simulink library "casper_library"  (Simulink 6.5)
PostLoadFcn:
  | % Stub definitions for mask variables
  | delay_depth=16;
  | n_bits=8;
  | bin_pt=7;
values from neighbouring files (symbols this model uses):
  add_latency = get_var('add_latency', 'defaults', defaults, varargin{:})    [butterfly_direct_init.m]    (also in fft_direct_init.m; fft_init.m; fft_wideband_real_init.m; pfb_real_add_tree_init.m)
  BitWidthIn = get_var('BitWidthIn', 'defaults', defaults, varargin{:})    [pfb_real_add_tree_init.m]
  blockCountBits = ceil(log2(numBlocks))    [address_gen_vacc_v2_mask.m]
  blockRowBits = 0    [address_gen_vacc_v2_mask.m]
  CoeffBitWidth = get_var('CoeffBitWidth', 'defaults', defaults, varargin{:})    [pfb_coeff_gen_init.m]    (also in pfb_real_add_tree_init.m)
  mult_latency = get_var('mult_latency', 'defaults', defaults, varargin{:})    [butterfly_direct_init.m]    (also in fft_direct_init.m; fft_init.m; fft_wideband_real_init.m)
  n_inputs = get_var('n_inputs', 'defaults', defaults, varargin{:})    [fft_init.m]    (also in fft_unscrambler_init.m; fft_wideband_real_init.m; partial_delay_init.m = get_var('n_inputs', varargin{:}); pfb_coeff_gen_init.m)
  PFBSize = get_var('PFBSize', 'defaults', defaults, varargin{:})    [pfb_coeff_gen_init.m]
undefined symbols (not defined in the file or in its folder): acc_len, ant_bits, bit_growth, cmult_4bit_br, cmult_4bit_em, cmult_4bit_sl, n_ants, n_bits_out, num_ants
libraries: xbsIndex_r3 x1646, xbsIndex_r4 x226, casper_library x156, xbsReplacements_r4 x17, xps_library x10, fft_library x4
(part 7 of 14)

== system casper_library/Correlator/x_engine_reorder/win2_ctrl ==
  write : Inport
  win_valid : Inport  Port=2
  sync : Inport  Port=3
  Constant : xbsIndex_r3/Constant  const=num_elements  equ=P=C  arith_type=Unsigned  n_bits=elements_bits + 1  bin_pt=0  opselect=C  inp2=PCIN>>17  opr=+  inp1=P  carry=CIN  iostate=0  explicit_period=on  period=1  dbl_ovrd=off
  Constant1 : xbsIndex_r3/Constant  const=num_elements * 2 - 2  equ=P=C  arith_type=Unsigned  n_bits=elements_bits + 1  bin_pt=0  opselect=C  inp2=PCIN>>17  opr=+  inp1=P  carry=CIN  iostate=0  explicit_period=on  period=1  dbl_ovrd=off
  Constant3 : xbsIndex_r3/Constant  const=num_elements * 2 - 1  equ=P=C  arith_type=Unsigned  n_bits=elements_bits + 1  bin_pt=0  opselect=C  inp2=PCIN>>17  opr=+  inp1=P  carry=CIN  iostate=0  explicit_period=on  period=1  dbl_ovrd=off
  Constant6 : xbsIndex_r3/Constant  const=num_elements  equ=P=C  arith_type=Unsigned  n_bits=elements_bits + 1  bin_pt=0  opselect=C  inp2=PCIN>>17  opr=+  inp1=P  carry=CIN  iostate=0  explicit_period=on  period=1  dbl_ovrd=off
  Counter : xbsIndex_r3/Counter  cnt_type=Free Running  n_bits=elements_bits + 1  bin_pt=0  arith_type=Unsigned  start_count=num_elements * 2 - 1 - addr_offset  cnt_to=71  cnt_by_val=1  operation=Up  explicit_period=off  period=1  load_pin=on  rst=on  en=on  dbl_ovrd=off  show_param=off  use_rpm=on  gen_core=off
      settings: xl_area=[0, 0, 0, 0, 0, 0, 0]
  Delay10 : xbsIndex_r3/Delay  latency=1  reg_retiming=off  explicit_period=off  period=1  en=on  accept_only_valid=off  init_zero=on  dbl_ovrd=off  show_param=off
      settings: xl_area=[0, 0, 0, 0, 0, 0, 0]
  Delay12 : xbsIndex_r3/Delay  latency=1  reg_retiming=off  explicit_period=off  period=1  en=on  accept_only_valid=off  init_zero=on  dbl_ovrd=off  show_param=off
      settings: xl_area=[0, 0, 0, 0, 0, 0, 0]
  Logical3 : xbsIndex_r3/Logical  logical_function=AND  inputs=2  precision=Full  arith_type=Unsigned  n_bits=8  bin_pt=2  align_bp=on  latency=0  explicit_period=off  period=1  en=off  dbl_ovrd=off  show_param=off
      settings: xl_area=[0, 0, 0, 0, 0, 0, 0]
  Logical6 : xbsIndex_r3/Logical  logical_function=AND  inputs=2  precision=Full  arith_type=Unsigned  n_bits=8  bin_pt=2  align_bp=on  latency=0  explicit_period=off  period=1  en=off  dbl_ovrd=off  show_param=off
      settings: xl_area=[0, 0, 0, 0, 0, 0, 0]
  Relational : xbsIndex_r3/Relational  mode=a>=b  latency=1  explicit_period=on  period=1  en=off  dbl_ovrd=off  show_param=off
      settings: xl_area=[0, 0, 0, 0, 0, 0, 0]
  Relational2 : xbsIndex_r3/Relational  mode=a=b  latency=1  explicit_period=on  period=1  en=off  dbl_ovrd=off  show_param=off
      settings: xl_area=[0, 0, 0, 0, 0, 0, 0]
  Relational4 : xbsIndex_r3/Relational  mode=a=b  latency=1  explicit_period=on  period=1  en=off  dbl_ovrd=off  show_param=off
      settings: xl_area=[0, 0, 0, 0, 0, 0, 0]
  pulse_extender1 : Subsystem  mask{num_elements=num_elements}
      mask prompts: num_elements "Length of Pulse"
      mask init:
      | pulse_len = 2*num_elements;
      | bits = ceil(log2(pulse_len));
  write_addr : Outport
  read : Outport  Port=2
  read_valid : Outport  Port=3
  wires:
  Constant/1 -> Counter/2
  Constant1/1 -> Relational/2
  Counter/1 -> Relational/1, Relational2/1, Relational4/1, write_addr/1
  Relational/1 -> Counter/1
  pulse_extender1/1(out) -> Logical6/1, read/1
  Constant3/1 -> Relational2/2
  Relational2/1 -> pulse_extender1/1(in), Delay12/2
  Constant6/1 -> Relational4/2
  Relational4/1 -> Logical3/1
  Logical3/1 -> Delay10/2
  Delay10/1 -> Delay12/1
  Delay12/1 -> Logical6/2
  sync/1 -> Counter/3
  win_valid/1 -> Delay10/1
  write/1 -> Counter/4, Logical3/2
  Logical6/1 -> read_valid/1

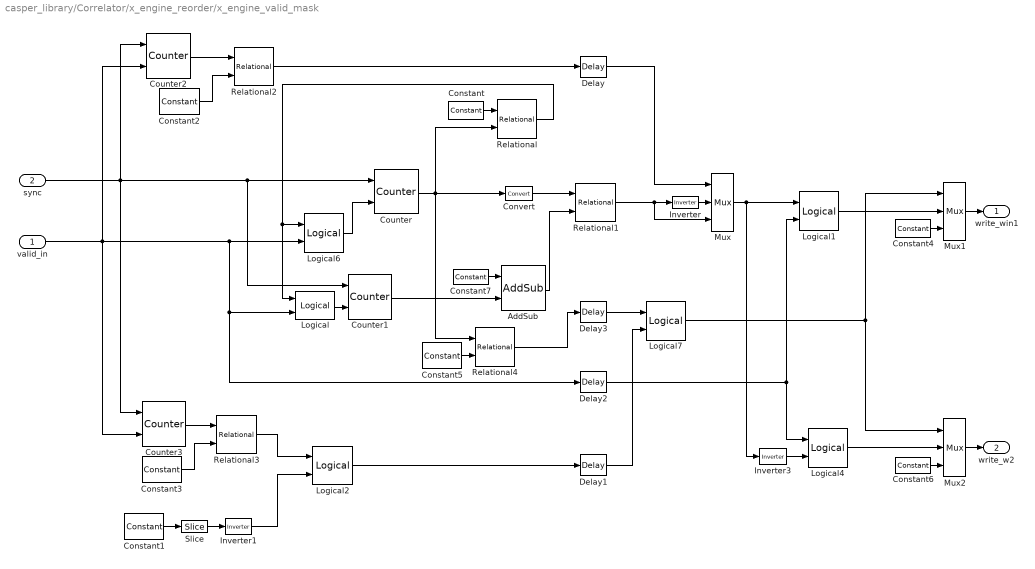
== system casper_library/Correlator/x_engine_reorder/x_engine_valid_mask ==
  valid_in : Inport
  sync : Inport  Port=2
  AddSub : xbsIndex_r3/AddSub  mode=Subtraction  precision=Full  arith_type=Unsigned  n_bits=8  bin_pt=2  quantization=Truncate  overflow=Wrap  latency=0  explicit_period=off  period=1  use_carryin=off  use_carryout=off  en=off  dbl_ovrd=off  show_param=off  use_core=on  pipeline=off  use_rpm=on  gen_core=off
      settings: xl_area=[0, 0, 0, 0, 0, 0, 0]
  Constant : xbsIndex_r3/Constant  const=num_taps-1  equ=P=C  arith_type=Unsigned  n_bits=cntr_bits  bin_pt=0  opselect=C  inp2=PCIN>>17  opr=+  inp1=P  carry=CIN  iostate=0  explicit_period=on  period=1  dbl_ovrd=off
  Constant1 : xbsIndex_r3/Constant  const=num_ants  equ=P=C  arith_type=Unsigned  n_bits=ant_bits  bin_pt=0  opselect=C  inp2=PCIN>>17  opr=+  inp1=P  carry=CIN  iostate=0  explicit_period=on  period=1  dbl_ovrd=off
  Constant2 : xbsIndex_r3/Constant  const=num_validins  equ=P=C  arith_type=Unsigned  n_bits=validin_bits  bin_pt=0  opselect=C  inp2=PCIN>>17  opr=+  inp1=P  carry=CIN  iostate=0  explicit_period=on  period=1  dbl_ovrd=off
  Constant3 : xbsIndex_r3/Constant  const=num_validins/2  equ=P=C  arith_type=Unsigned  n_bits=validin_bits - 1  bin_pt=0  opselect=C  inp2=PCIN>>17  opr=+  inp1=P  carry=CIN  iostate=0  explicit_period=on  period=1  dbl_ovrd=off
  Constant4 : xbsIndex_r3/Constant  const=0  equ=P=C  arith_type=Boolean  n_bits=1  bin_pt=0  opselect=C  inp2=PCIN>>17  opr=+  inp1=P  carry=CIN  iostate=0  explicit_period=on  period=1  dbl_ovrd=off
  Constant5 : xbsIndex_r3/Constant  const=0  equ=P=C  arith_type=Unsigned  n_bits=cntr_bits  bin_pt=0  opselect=C  inp2=PCIN>>17  opr=+  inp1=P  carry=CIN  iostate=0  explicit_period=on  period=1  dbl_ovrd=off
  Constant6 : xbsIndex_r3/Constant  const=0  equ=P=C  arith_type=Boolean  n_bits=1  bin_pt=0  opselect=C  inp2=PCIN>>17  opr=+  inp1=P  carry=CIN  iostate=0  explicit_period=on  period=1  dbl_ovrd=off
  Constant7 : xbsIndex_r3/Constant  const=num_taps-1  equ=P=C  arith_type=Unsigned  n_bits=cntr_bits  bin_pt=0  opselect=C  inp2=PCIN>>17  opr=+  inp1=P  carry=CIN  iostate=0  explicit_period=on  period=1  dbl_ovrd=off
  Convert : xbsIndex_r3/Convert  arith_type=Unsigned  n_bits=cntr_bits+1  bin_pt=0  quantization=Truncate  overflow=Wrap  latency=0  explicit_period=off  period=1  dbl_ovrd=off  show_param=off  inserted_by_tool=off  pipeline=off
      settings: xl_area=[0, 0, 0, 0, 0, 0, 0]
  Counter : xbsIndex_r3/Counter  cnt_type=Count Limited  n_bits=cntr_bits  bin_pt=0  arith_type=Unsigned  start_count=0  cnt_to=num_taps-1  cnt_by_val=1  operation=Up  explicit_period=off  period=1  load_pin=off  rst=on  en=on  dbl_ovrd=off  show_param=off  use_rpm=on  gen_core=off
      settings: xl_area=[0, 0, 0, 0, 0, 0, 0]
  Counter1 : xbsIndex_r3/Counter  cnt_type=Count Limited  n_bits=ant_bits  bin_pt=0  arith_type=Unsigned  start_count=0  cnt_to=num_ants-1  cnt_by_val=1  operation=Up  explicit_period=off  period=1  load_pin=off  rst=on  en=on  dbl_ovrd=off  show_param=off  use_rpm=on  gen_core=off
      settings: xl_area=[0, 0, 0, 0, 0, 0, 0]
  Counter2 : xbsIndex_r3/Counter  cnt_type=Count Limited  n_bits=validin_bits + 1  bin_pt=0  arith_type=Unsigned  start_count=1  cnt_to=num_validins * 2  cnt_by_val=1  operation=Up  explicit_period=off  period=1  load_pin=off  rst=on  en=on  dbl_ovrd=off  show_param=off  use_rpm=on  gen_core=off
      settings: xl_area=[0, 0, 0, 0, 0, 0, 0]
  Counter3 : xbsIndex_r3/Counter  cnt_type=Count Limited  n_bits=validin_bits  bin_pt=0  arith_type=Unsigned  start_count=1  cnt_to=num_validins  cnt_by_val=1  operation=Up  explicit_period=off  period=1  load_pin=off  rst=on  en=on  dbl_ovrd=off  show_param=off  use_rpm=on  gen_core=off
      settings: xl_area=[0, 0, 0, 0, 0, 0, 0]
  Delay{,1..3} (4 alike) : xbsIndex_r3/Delay  latency=1  reg_retiming=off  explicit_period=off  period=1  en=off  accept_only_valid=off  init_zero=on  dbl_ovrd=off  show_param=off
      settings: xl_area=[0, 0, 0, 0, 0, 0, 0]
  Inverter : xbsIndex_r3/Inverter  latency=0  explicit_period=off  period=1  en=off  dbl_ovrd=off  show_param=off
      settings: xl_area=[0, 0, 0, 0, 0, 0, 0]
  Inverter1 : xbsIndex_r3/Inverter  latency=0  explicit_period=off  period=1  en=off  dbl_ovrd=off  show_param=off
      settings: xl_area=[0, 0, 0, 0, 0, 0, 0]
  Inverter3 : xbsIndex_r3/Inverter  latency=0  explicit_period=off  period=1  en=off  dbl_ovrd=off  show_param=off
      settings: xl_area=[0, 0, 0, 0, 0, 0, 0]
  Logical{,1..2,4,7} (5 alike) : xbsIndex_r3/Logical  logical_function=AND  inputs=2  precision=Full  arith_type=Unsigned  n_bits=8  bin_pt=2  align_bp=on  latency=0  explicit_period=off  period=1  en=off  dbl_ovrd=off  show_param=off
      settings: xl_area=[0, 0, 0, 0, 0, 0, 0]
  Logical6 : xbsIndex_r3/Logical  logical_function=OR  inputs=2  precision=Full  arith_type=Unsigned  n_bits=8  bin_pt=2  align_bp=on  latency=0  explicit_period=off  period=1  en=off  dbl_ovrd=off  show_param=off
      settings: xl_area=[0, 0, 0, 0, 0, 0, 0]
  Mux : xbsIndex_r3/Mux  inputs=2  precision=Full  arith_type="Signed  (2's comp)"  n_bits=8  bin_pt=2  quantization=Truncate  overflow=Wrap  latency=0  explicit_period=off  period=1  en=off  dbl_ovrd=off  show_param=off  mux_type=off  use_rpm=off  gen_core=off
      settings: xl_area=[0, 0, 0, 0, 0, 0, 0]
  Mux1 : xbsIndex_r3/Mux  inputs=2  precision=Full  arith_type="Signed  (2's comp)"  n_bits=8  bin_pt=2  quantization=Truncate  overflow=Wrap  latency=0  explicit_period=off  period=1  en=off  dbl_ovrd=off  show_param=off  mux_type=off  use_rpm=off  gen_core=off
      settings: xl_area=[0, 0, 0, 0, 0, 0, 0]
  Mux2 : xbsIndex_r3/Mux  inputs=2  precision=Full  arith_type="Signed  (2's comp)"  n_bits=8  bin_pt=2  quantization=Truncate  overflow=Wrap  latency=0  explicit_period=off  period=1  en=off  dbl_ovrd=off  show_param=off  mux_type=off  use_rpm=off  gen_core=off
      settings: xl_area=[0, 0, 0, 0, 0, 0, 0]
  Relational : xbsIndex_r3/Relational  mode=a=b  latency=0  explicit_period=on  period=1  en=off  dbl_ovrd=off  show_param=off
      settings: xl_area=[0, 0, 0, 0, 0, 0, 0]
  Relational1 : xbsIndex_r3/Relational  mode=a>=b  latency=1  explicit_period=off  period=1  en=off  dbl_ovrd=off  show_param=off
      settings: xl_area=[0, 0, 0, 0, 0, 0, 0]
  Relational2 : xbsIndex_r3/Relational  mode=a<=b  latency=0  explicit_period=off  period=1  en=off  dbl_ovrd=off  show_param=off
      settings: xl_area=[0, 0, 0, 0, 0, 0, 0]
  Relational3 : xbsIndex_r3/Relational  mode=a<b  latency=0  explicit_period=off  period=1  en=off  dbl_ovrd=off  show_param=off
      settings: xl_area=[0, 0, 0, 0, 0, 0, 0]
  Relational4 : xbsIndex_r3/Relational  mode=a=b  latency=0  explicit_period=on  period=1  en=off  dbl_ovrd=off  show_param=off
      settings: xl_area=[0, 0, 0, 0, 0, 0, 0]
  Slice : xbsIndex_r3/Slice  mode=Lower Bit Location + Width  nbits=1  bit1=0  base1=MSB of Input  bit0=0  base0=LSB of Input  boolean_output=on  explicit_period=off  period=1  dbl_ovrd=off
  write_win1 : Outport
  write_w2 : Outport  Port=2
  wires:
  Counter/1 -> Relational/2, Convert/1, Relational4/1
  AddSub/1 -> Relational1/2
  Constant/1 -> Relational/1
  Relational/1 -> Logical/1, Logical6/1
  Relational1/1 -> Mux/3, Inverter/1
  Mux/1 -> Logical1/1, Inverter3/1
  sync/1 -> Counter2/1, Counter/1, Counter1/1, Counter3/1
  valid_in/1 -> Counter2/2, Logical/2, Delay2/1, Logical6/2, Counter3/2
  Delay/1 -> Mux/1
  Convert/1 -> Relational1/1
  Inverter/1 -> Mux/2
  Delay2/1 -> Logical1/2, Logical4/1
  Logical1/1 -> Mux1/2
  Inverter3/1 -> Logical4/2
  Logical4/1 -> Mux2/2
  Logical7/1 -> Mux2/1, Mux1/1
  Mux1/1 -> write_win1/1
  Mux2/1 -> write_w2/1
  Counter1/1 -> AddSub/2
  Logical/1 -> Counter1/2
  Counter2/1 -> Relational2/1
  Relational2/1 -> Delay/1
  Constant2/1 -> Relational2/2
  Counter3/1 -> Relational3/1
  Constant3/1 -> Relational3/2
  Delay1/1 -> Logical7/2
  Constant4/1 -> Mux1/3
  Constant1/1 -> Slice/1
  Slice/1 -> Inverter1/1
  Relational3/1 -> Logical2/1
  Inverter1/1 -> Logical2/2
  Logical2/1 -> Delay1/1
  Delay3/1 -> Logical7/1
  Logical6/1 -> Counter/2
  Relational4/1 -> Delay3/1
  Constant5/1 -> Relational4/2
  Constant6/1 -> Mux2/3
  Constant7/1 -> AddSub/1

== system casper_library/Delays/delay_complex/delay1 ==
  In1 : Inport
  delay_bram : casper_library/Delays/delay_bram  DelayLen=delay  bram_latency=bram_latency
  Out1 : Outport
  wires:
  In1/1 -> delay_bram/1
  delay_bram/1 -> Out1/1

== system casper_library/Delays/delay_complex/delay2 ==
  In1 : Inport
  delay_bram : casper_library/Delays/delay_bram  DelayLen=delay  bram_latency=bram_latency
  Out1 : Outport
  wires:
  In1/1 -> delay_bram/1
  delay_bram/1 -> Out1/1

== system casper_library/Downconverter/dec_fir/fir_col1 ==
  real1 : Inport
  imag1 : Inport  Port=2
  real2 : Inport  Port=3
  imag2 : Inport  Port=4
  adder_tree1 : Subsystem  AncestorBlock=casper_library/Misc/adder_tree  mask(adder_tree){n_inputs=2, latency=2}
      mask prompts: n_inputs "Number of Inputs"; latency "Add Latency"
      mask help: Sums all inputs using a tree of adds and delays.
      mask init:
      | adder_tree_init(gcb, ...
      |     'n_inputs', n_inputs, ...
      |     'latency', latency);
      settings: AttributesFormatString=latency 2
      mask Help: eval('xlWeb([getenv(''MLIB_ROOT''), ''\doc\html\sp_adder_tree\sp_adder_tree.html''])')
  adder_tree2 : Subsystem  AncestorBlock=casper_library/Misc/adder_tree  mask(adder_tree){n_inputs=2, latency=2}
      mask prompts: n_inputs "Number of Inputs"; latency "Add Latency"
      mask help: Sums all inputs using a tree of adds and delays.
      mask init:
      | adder_tree_init(gcb, ...
      |     'n_inputs', n_inputs, ...
      |     'latency', latency);
      settings: AttributesFormatString=latency 2
      mask Help: eval('xlWeb([getenv(''MLIB_ROOT''), ''\doc\html\sp_adder_tree\sp_adder_tree.html''])')
  c1 : xbsIndex_r4/Constant  arith_type=Unsigned  const=1  n_bits=1  bin_pt=0  explicit_period=on  period=1  equ=P=C  opselect=C  inp2=PCIN>>17  opr=+  inp1=P  carry=CIN  dbl_ovrd=off  block_type=constant
      settings: block_version=9.1.01
  c2 : xbsIndex_r4/Constant  arith_type=Unsigned  const=1  n_bits=1  bin_pt=0  explicit_period=on  period=1  equ=P=C  opselect=C  inp2=PCIN>>17  opr=+  inp1=P  carry=CIN  dbl_ovrd=off  block_type=constant
      settings: block_version=9.1.01
  fir_tap1 : casper_library/Downconverter/fir_tap  SystemSampleTime=-1  factor=5  latency=45
  fir_tap2 : casper_library/Downconverter/fir_tap  SystemSampleTime=-1  factor=4  latency=45
  real_out1 : Outport
  imag_out1 : Outport  Port=2
  real_out2 : Outport  Port=3
  imag_out2 : Outport  Port=4
  real_sum : Outport  Port=5
  imag_sum : Outport  Port=6
  wires:
  fir_tap2/4 -> adder_tree2/3(din2)
  fir_tap2/3 -> adder_tree1/3(din2)
  fir_tap2/2 -> imag_out2/1
  fir_tap2/1 -> real_out2/1
  imag2/1 -> fir_tap2/2
  real2/1 -> fir_tap2/1
  fir_tap1/4 -> adder_tree2/2(din1)
  fir_tap1/3 -> adder_tree1/2(din1)
  fir_tap1/2 -> imag_out1/1
  fir_tap1/1 -> real_out1/1
  imag1/1 -> fir_tap1/2
  real1/1 -> fir_tap1/1
  adder_tree2/2(dout) -> imag_sum/1
  adder_tree1/2(dout) -> real_sum/1
  c2/1 -> adder_tree2/1(sync)
  c1/1 -> adder_tree1/1(sync)

== system casper_library/Downconverter/dec_fir/imag_sum ==
  sync : Inport
  din1 : Inport  Port=2
  sync_delay : xbsIndex_r4/Delay  en=off  latency=0  dbl_ovrd=off  reg_retiming=off  block_type=delay
      settings: xl_area=[0, 0, 0, 0, 0, 0, 0]  block_version=9.1.01
  sync_out : Outport
  dout : Outport  Port=2
  wires:
  din1/1 -> dout/1
  sync_delay/1 -> sync_out/1
  sync/1 -> sync_delay/1

== system casper_library/Downconverter/dec_fir/real_sum ==
  sync : Inport
  din1 : Inport  Port=2
  sync_delay : xbsIndex_r4/Delay  en=off  latency=0  dbl_ovrd=off  reg_retiming=off  block_type=delay
      settings: xl_area=[0, 0, 0, 0, 0, 0, 0]  block_version=9.1.01
  sync_out : Outport
  dout : Outport  Port=2
  wires:
  din1/1 -> dout/1
  sync_delay/1 -> sync_out/1
  sync/1 -> sync_delay/1

== system casper_library/Downconverter/dec_fir/ri_to_c ==
  re : Inport
  im : Inport  Port=2
  Concat : xbsIndex_r4/Concat  num_inputs=2  dbl_ovrd=off  block_type=concat
      settings: block_version=9.1.01
  Reinterpret : xbsIndex_r4/Reinterpret  force_arith_type=on  arith_type=Unsigned  force_bin_pt=on  bin_pt=0  block_type=reinterpret
      settings: infoedit="Changes signal type without altering the binary representation.   You can changed the signal between signed and unsigned, and relocate the binary point.<P><P>Hardware notes: In hardware this block costs nothing.<P><P>Example:  Suppose the input is 6 bits wide, signed, with 2 fractional bits, and the output is forced to unsigned with 0 fractional bits.  Then an input of -2.0 (1110.00 in binary 2's complement) becomes an output of 56 (111000 in binary)."  block_version=9.1.01
  Reinterpret1 : xbsIndex_r4/Reinterpret  force_arith_type=on  arith_type=Unsigned  force_bin_pt=on  bin_pt=0  block_type=reinterpret
      settings: infoedit="Changes signal type without altering the binary representation.   You can changed the signal between signed and unsigned, and relocate the binary point.<P><P>Hardware notes: In hardware this block costs nothing.<P><P>Example:  Suppose the input is 6 bits wide, signed, with 2 fractional bits, and the output is forced to unsigned with 0 fractional bits.  Then an input of -2.0 (1110.00 in binary 2's complement) becomes an output of 56 (111000 in binary)."  block_version=9.1.01
  c : Outport
  wires:
  Reinterpret/1 -> Concat/1
  Reinterpret1/1 -> Concat/2
  re/1 -> Reinterpret/1
  Concat/1 -> c/1
  im/1 -> Reinterpret1/1

== system casper_library/Downconverter/fir_col/adder_tree1 ==
  sync : Inport
  din1 : Inport  Port=2
  din2 : Inport  Port=3
  addr1 : xbsIndex_r4/AddSub  mode=Addition  use_carryin=off  use_carryout=off  en=off  latency=3  precision=Full  arith_type=Unsigned  n_bits=8  bin_pt=2  quantization=Truncate  overflow=Wrap  dbl_ovrd=off  use_behavioral_HDL=on  pipelined=on  use_rpm=on  block_type=addsub
      settings: xl_area=[0, 0, 0, 0, 0, 0, 0]  block_version=9.1.01
  sync_delay : xbsIndex_r4/Delay  en=off  latency=3  dbl_ovrd=off  reg_retiming=off  block_type=delay
      settings: xl_area=[0, 0, 0, 0, 0, 0, 0]  block_version=9.1.01
  sync_out : Outport
  dout : Outport  Port=2
  wires:
  addr1/1 -> dout/1
  din2/1 -> addr1/2
  din1/1 -> addr1/1
  sync_delay/1 -> sync_out/1
  sync/1 -> sync_delay/1

== system casper_library/Downconverter/fir_col/adder_tree2 ==
  sync : Inport
  din1 : Inport  Port=2
  din2 : Inport  Port=3
  addr1 : xbsIndex_r4/AddSub  mode=Addition  use_carryin=off  use_carryout=off  en=off  latency=3  precision=Full  arith_type=Unsigned  n_bits=8  bin_pt=2  quantization=Truncate  overflow=Wrap  dbl_ovrd=off  use_behavioral_HDL=on  pipelined=on  use_rpm=on  block_type=addsub
      settings: xl_area=[0, 0, 0, 0, 0, 0, 0]  block_version=9.1.01
  sync_delay : xbsIndex_r4/Delay  en=off  latency=3  dbl_ovrd=off  reg_retiming=off  block_type=delay
      settings: xl_area=[0, 0, 0, 0, 0, 0, 0]  block_version=9.1.01
  sync_out : Outport
  dout : Outport  Port=2
  wires:
  addr1/1 -> dout/1
  din2/1 -> addr1/2
  din1/1 -> addr1/1
  sync_delay/1 -> sync_out/1
  sync/1 -> sync_delay/1

== system casper_library/Downconverter/fir_col/fir_tap1 ==
  a : Inport
  b : Inport  Port=2
  Constant : xbsIndex_r4/Constant  arith_type=Signed (2's comp)  const=factor  n_bits=18  bin_pt=17  explicit_period=on  period=1  equ=P=C  opselect=C  inp2=PCIN>>17  opr=+  inp1=P  carry=CIN  dbl_ovrd=off  block_type=constant
      settings: block_version=9.1.01
  Mult : xbsIndex_r4/Mult  precision=Full  arith_type="Signed  (2's comp)"  n_bits=18  bin_pt=17  quantization=Truncate  overflow=Wrap  en=off  latency=latency  dbl_ovrd=off  use_behavioral_HDL=off  use_embedded=on  opt=Speed  optimum_pipeline=off  pipeline=on  use_rpm=off  placement_style=Rectangular shape  block_type=mult
      settings: infoedit=Hardware notes: To use the internal pipeline stage of the dedicated multiplier you must select 'Pipeline for maximum performance'.  xl_area=[0, 0, 0, 0, 0, 0, 0]  block_version=9.1.01
  Mult1 : xbsIndex_r4/Mult  precision=Full  arith_type="Signed  (2's comp)"  n_bits=18  bin_pt=17  quantization=Truncate  overflow=Wrap  en=off  latency=latency  dbl_ovrd=off  use_behavioral_HDL=off  use_embedded=on  opt=Speed  optimum_pipeline=off  pipeline=on  use_rpm=off  placement_style=Rectangular shape  block_type=mult
      settings: infoedit=Hardware notes: To use the internal pipeline stage of the dedicated multiplier you must select 'Pipeline for maximum performance'.  xl_area=[0, 0, 0, 0, 0, 0, 0]  block_version=9.1.01
  Register : xbsIndex_r4/Register  init=0  rst=off  en=off  dbl_ovrd=off  block_type=register
      settings: xl_area=[0, 0, 0, 0, 0, 0, 0]  block_version=9.1.01
  Register1 : xbsIndex_r4/Register  init=0  rst=off  en=off  dbl_ovrd=off  block_type=register
      settings: xl_area=[0, 0, 0, 0, 0, 0, 0]  block_version=9.1.01
  warn period Mult0 : xbsReplacements_r4/Warning  SystemSampleTime=-1  period=1
  warn period Mult10 : xbsReplacements_r4/Warning  SystemSampleTime=-1  period=1
  warn period Register0 : xbsReplacements_r4/Warning  SystemSampleTime=-1  period=1
  warn period Register10 : xbsReplacements_r4/Warning  SystemSampleTime=-1  period=1
  a_out : Outport
  b_out : Outport  Port=2
  real : Outport  Port=3
  imag : Outport  Port=4
  wires:
  Mult1/1 -> real/1
  b/1 -> Mult/2, Register1/1
  Mult/1 -> imag/1
  a/1 -> Mult1/2, Register/1
  Constant/1 -> Mult1/1, Mult/1
  Register/1 -> a_out/1
  Register1/1 -> b_out/1

== system casper_library/Downconverter/fir_col/fir_tap2 ==
  a : Inport
  b : Inport  Port=2
  Constant : xbsIndex_r4/Constant  arith_type=Signed (2's comp)  const=factor  n_bits=18  bin_pt=17  explicit_period=on  period=1  equ=P=C  opselect=C  inp2=PCIN>>17  opr=+  inp1=P  carry=CIN  dbl_ovrd=off  block_type=constant
      settings: block_version=9.1.01
  Mult : xbsIndex_r4/Mult  precision=Full  arith_type="Signed  (2's comp)"  n_bits=18  bin_pt=17  quantization=Truncate  overflow=Wrap  en=off  latency=latency  dbl_ovrd=off  use_behavioral_HDL=off  use_embedded=on  opt=Speed  optimum_pipeline=off  pipeline=on  use_rpm=off  placement_style=Rectangular shape  block_type=mult
      settings: infoedit=Hardware notes: To use the internal pipeline stage of the dedicated multiplier you must select 'Pipeline for maximum performance'.  xl_area=[0, 0, 0, 0, 0, 0, 0]  block_version=9.1.01
  Mult1 : xbsIndex_r4/Mult  precision=Full  arith_type="Signed  (2's comp)"  n_bits=18  bin_pt=17  quantization=Truncate  overflow=Wrap  en=off  latency=latency  dbl_ovrd=off  use_behavioral_HDL=off  use_embedded=on  opt=Speed  optimum_pipeline=off  pipeline=on  use_rpm=off  placement_style=Rectangular shape  block_type=mult
      settings: infoedit=Hardware notes: To use the internal pipeline stage of the dedicated multiplier you must select 'Pipeline for maximum performance'.  xl_area=[0, 0, 0, 0, 0, 0, 0]  block_version=9.1.01
  Register : xbsIndex_r4/Register  init=0  rst=off  en=off  dbl_ovrd=off  block_type=register
      settings: xl_area=[0, 0, 0, 0, 0, 0, 0]  block_version=9.1.01
  Register1 : xbsIndex_r4/Register  init=0  rst=off  en=off  dbl_ovrd=off  block_type=register
      settings: xl_area=[0, 0, 0, 0, 0, 0, 0]  block_version=9.1.01
  warn period Mult0 : xbsReplacements_r4/Warning  SystemSampleTime=-1  period=1
  warn period Mult10 : xbsReplacements_r4/Warning  SystemSampleTime=-1  period=1
  warn period Register0 : xbsReplacements_r4/Warning  SystemSampleTime=-1  period=1
  warn period Register10 : xbsReplacements_r4/Warning  SystemSampleTime=-1  period=1
  a_out : Outport
  b_out : Outport  Port=2
  real : Outport  Port=3
  imag : Outport  Port=4
  wires:
  Mult1/1 -> real/1
  b/1 -> Mult/2, Register1/1
  Mult/1 -> imag/1
  a/1 -> Mult1/2, Register/1
  Constant/1 -> Mult1/1, Mult/1
  Register/1 -> a_out/1
  Register1/1 -> b_out/1

== system casper_library/Downconverter/fir_dbl_col/adder_tree1 ==
  sync : Inport
  din1 : Inport  Port=2
  din2 : Inport  Port=3
  addr1 : xbsIndex_r3/AddSub  mode=Addition  precision=Full  arith_type=Unsigned  n_bits=8  bin_pt=2  quantization=Truncate  overflow=Wrap  latency=1  explicit_period=on  period=1  use_carryin=off  use_carryout=off  en=off  dbl_ovrd=off  show_param=off  use_core=on  pipeline=on  use_rpm=on  gen_core=off
      settings: xl_area=[0, 0, 0, 0, 0, 0, 0]
  sync_delay : xbsIndex_r3/Delay  latency=1  reg_retiming=off  explicit_period=off  period=1  en=off  accept_only_valid=off  init_zero=on  dbl_ovrd=off  show_param=off
      settings: xl_area=[0, 0, 0, 0, 0, 0, 0]
  sync_out : Outport
  dout : Outport  Port=2
  wires:
  addr1/1 -> dout/1
  din2/1 -> addr1/2
  din1/1 -> addr1/1
  sync_delay/1 -> sync_out/1
  sync/1 -> sync_delay/1

== system casper_library/Downconverter/fir_dbl_col/adder_tree2 ==
  sync : Inport
  din1 : Inport  Port=2
  din2 : Inport  Port=3
  addr1 : xbsIndex_r3/AddSub  mode=Addition  precision=Full  arith_type=Unsigned  n_bits=8  bin_pt=2  quantization=Truncate  overflow=Wrap  latency=1  explicit_period=on  period=1  use_carryin=off  use_carryout=off  en=off  dbl_ovrd=off  show_param=off  use_core=on  pipeline=on  use_rpm=on  gen_core=off
      settings: xl_area=[0, 0, 0, 0, 0, 0, 0]
  sync_delay : xbsIndex_r3/Delay  latency=1  reg_retiming=off  explicit_period=off  period=1  en=off  accept_only_valid=off  init_zero=on  dbl_ovrd=off  show_param=off
      settings: xl_area=[0, 0, 0, 0, 0, 0, 0]
  sync_out : Outport
  dout : Outport  Port=2
  wires:
  addr1/1 -> dout/1
  din2/1 -> addr1/2
  din1/1 -> addr1/1
  sync_delay/1 -> sync_out/1
  sync/1 -> sync_delay/1

== system casper_library/Downconverter/fir_dbl_col/fir_dbl_tap1 ==
  a : Inport
  b : Inport  Port=2
  c : Inport  Port=3
  d : Inport  Port=4
  AddSub : xbsIndex_r3/AddSub  mode=Addition  precision=User Defined  arith_type="Signed  (2's comp)"  n_bits=18  bin_pt=16  quantization=Truncate  overflow=Wrap  latency=add_latency  explicit_period=on  period=1  use_carryin=off  use_carryout=off  en=off  dbl_ovrd=off  show_param=off  use_core=on  pipeline=off  use_rpm=on  gen_core=off
      settings: xl_area=[0, 0, 0, 0, 0, 0, 0]
  AddSub1 : xbsIndex_r3/AddSub  mode=Addition  precision=User Defined  arith_type="Signed  (2's comp)"  n_bits=18  bin_pt=16  quantization=Truncate  overflow=Wrap  latency=add_latency  explicit_period=on  period=1  use_carryin=off  use_carryout=off  en=off  dbl_ovrd=off  show_param=off  use_core=on  pipeline=off  use_rpm=on  gen_core=off
      settings: xl_area=[0, 0, 0, 0, 0, 0, 0]
  Constant : xbsIndex_r3/Constant  const=factor  equ=P=C  arith_type="Signed  (2's comp)"  n_bits=18  bin_pt=17  opselect=C  inp2=PCIN>>17  opr=+  inp1=P  carry=CIN  iostate=0  explicit_period=on  period=1  dbl_ovrd=off
  Mult : xbsIndex_r3/Mult  precision=Full  arith_type="Signed  (2's comp)"  n_bits=18  bin_pt=17  quantization=Truncate  overflow=Wrap  latency=mult_latency  explicit_period=off  period=1  en=off  dbl_ovrd=off  show_param=on  mult_type=Parallel  oversample=2  use_embedded=on  pipeline=on  use_rpm=off  placement_style=Rectangular Shape  gen_core=off
      settings: xl_area=[0, 0, 0, 0, 0, 0, 0]
  Mult1 : xbsIndex_r3/Mult  precision=Full  arith_type="Signed  (2's comp)"  n_bits=18  bin_pt=17  quantization=Truncate  overflow=Wrap  latency=mult_latency  explicit_period=off  period=1  en=off  dbl_ovrd=off  show_param=on  mult_type=Parallel  oversample=2  use_embedded=on  pipeline=on  use_rpm=off  placement_style=Rectangular Shape  gen_core=off
      settings: xl_area=[0, 0, 0, 0, 0, 0, 0]
  Register{,1..3} (4 alike) : xbsIndex_r3/Register  init=0  reg_only_valid=off  explicit_period=on  period=1  rst=off  en=off  out_en=off  dbl_ovrd=off  show_param=off
      settings: xl_area=[0, 0, 0, 0, 0, 0, 0]
  a_out : Outport
  b_out : Outport  Port=2
  c_out : Outport  Port=3
  d_out : Outport  Port=4
  real : Outport  Port=5
  imag : Outport  Port=6
  wires:
  Register1/1 -> b_out/1
  Register/1 -> a_out/1
  Constant/1 -> Mult/1, Mult1/1
  Mult/1 -> imag/1
  Mult1/1 -> real/1
  Register3/1 -> d_out/1
  Register2/1 -> c_out/1
  a/1 -> Register/1, AddSub/1
  b/1 -> Register1/1, AddSub1/1
  c/1 -> Register2/1, AddSub/2
  d/1 -> Register3/1, AddSub1/2
  AddSub/1 -> Mult1/2
  AddSub1/1 -> Mult/2

== system casper_library/Downconverter/fir_dbl_col/fir_dbl_tap2 ==
  a : Inport
  b : Inport  Port=2
  c : Inport  Port=3
  d : Inport  Port=4
  AddSub : xbsIndex_r3/AddSub  mode=Addition  precision=User Defined  arith_type="Signed  (2's comp)"  n_bits=18  bin_pt=16  quantization=Truncate  overflow=Wrap  latency=add_latency  explicit_period=on  period=1  use_carryin=off  use_carryout=off  en=off  dbl_ovrd=off  show_param=off  use_core=on  pipeline=off  use_rpm=on  gen_core=off
      settings: xl_area=[0, 0, 0, 0, 0, 0, 0]
  AddSub1 : xbsIndex_r3/AddSub  mode=Addition  precision=User Defined  arith_type="Signed  (2's comp)"  n_bits=18  bin_pt=16  quantization=Truncate  overflow=Wrap  latency=add_latency  explicit_period=on  period=1  use_carryin=off  use_carryout=off  en=off  dbl_ovrd=off  show_param=off  use_core=on  pipeline=off  use_rpm=on  gen_core=off
      settings: xl_area=[0, 0, 0, 0, 0, 0, 0]
  Constant : xbsIndex_r3/Constant  const=factor  equ=P=C  arith_type="Signed  (2's comp)"  n_bits=18  bin_pt=17  opselect=C  inp2=PCIN>>17  opr=+  inp1=P  carry=CIN  iostate=0  explicit_period=on  period=1  dbl_ovrd=off
  Mult : xbsIndex_r3/Mult  precision=Full  arith_type="Signed  (2's comp)"  n_bits=18  bin_pt=17  quantization=Truncate  overflow=Wrap  latency=mult_latency  explicit_period=off  period=1  en=off  dbl_ovrd=off  show_param=on  mult_type=Parallel  oversample=2  use_embedded=on  pipeline=on  use_rpm=off  placement_style=Rectangular Shape  gen_core=off
      settings: xl_area=[0, 0, 0, 0, 0, 0, 0]
  Mult1 : xbsIndex_r3/Mult  precision=Full  arith_type="Signed  (2's comp)"  n_bits=18  bin_pt=17  quantization=Truncate  overflow=Wrap  latency=mult_latency  explicit_period=off  period=1  en=off  dbl_ovrd=off  show_param=on  mult_type=Parallel  oversample=2  use_embedded=on  pipeline=on  use_rpm=off  placement_style=Rectangular Shape  gen_core=off
      settings: xl_area=[0, 0, 0, 0, 0, 0, 0]
  Register{,1..3} (4 alike) : xbsIndex_r3/Register  init=0  reg_only_valid=off  explicit_period=on  period=1  rst=off  en=off  out_en=off  dbl_ovrd=off  show_param=off
      settings: xl_area=[0, 0, 0, 0, 0, 0, 0]
  a_out : Outport
  b_out : Outport  Port=2
  c_out : Outport  Port=3
  d_out : Outport  Port=4
  real : Outport  Port=5
  imag : Outport  Port=6
  wires:
  Register1/1 -> b_out/1
  Register/1 -> a_out/1
  Constant/1 -> Mult/1, Mult1/1
  Mult/1 -> imag/1
  Mult1/1 -> real/1
  Register3/1 -> d_out/1
  Register2/1 -> c_out/1
  a/1 -> Register/1, AddSub/1
  b/1 -> Register1/1, AddSub1/1
  c/1 -> Register2/1, AddSub/2
  d/1 -> Register3/1, AddSub1/2
  AddSub/1 -> Mult1/2
  AddSub1/1 -> Mult/2

== system casper_library/Downconverter/mixer/dds ==
  lo_const0 : casper_library/Downconverter/lo_const  SystemSampleTime=-1  n_bits=4  phase=0
  lo_const1 : casper_library/Downconverter/lo_const  SystemSampleTime=-1  n_bits=4  phase=6.2832
  sin0 : Outport
  cos0 : Outport  Port=2
  sin1 : Outport  Port=3
  cos1 : Outport  Port=4
  wires:
  lo_const1/2 -> cos1/1
  lo_const1/1 -> sin1/1
  lo_const0/2 -> cos0/1
  lo_const0/1 -> sin0/1

== system casper_library/Downconverter/mixer/rcmult1 ==
  d : Inport
  sin : Inport  Port=2
  cos : Inport  Port=3
  Mult : xbsIndex_r4/Mult  precision=Full  arith_type="Signed  (2's comp)"  n_bits=8  bin_pt=2  quantization=Truncate  overflow=Wrap  en=off  latency=latency  dbl_ovrd=off  use_behavioral_HDL=off  use_embedded=on  opt=Speed  optimum_pipeline=off  pipeline=on  use_rpm=off  placement_style=Rectangular shape  block_type=mult
      settings: infoedit=Hardware notes: To use the internal pipeline stage of the dedicated multiplier you must select 'Pipeline for maximum performance'.  xl_area=[0, 0, 0, 0, 0, 0, 0]  block_version=9.1.01
  Mult1 : xbsIndex_r4/Mult  precision=Full  arith_type="Signed  (2's comp)"  n_bits=8  bin_pt=2  quantization=Truncate  overflow=Wrap  en=off  latency=latency  dbl_ovrd=off  use_behavioral_HDL=off  use_embedded=on  opt=Speed  optimum_pipeline=off  pipeline=on  use_rpm=off  placement_style=Rectangular shape  block_type=mult
      settings: infoedit=Hardware notes: To use the internal pipeline stage of the dedicated multiplier you must select 'Pipeline for maximum performance'.  xl_area=[0, 0, 0, 0, 0, 0, 0]  block_version=9.1.01
  real : Outport
  imag : Outport  Port=2
  wires:
  cos/1 -> Mult/2
  sin/1 -> Mult1/2
  d/1 -> Mult/1, Mult1/1
  Mult/1 -> real/1
  Mult1/1 -> imag/1

== system casper_library/Downconverter/mixer/rcmult2 ==
  d : Inport
  sin : Inport  Port=2
  cos : Inport  Port=3
  Mult : xbsIndex_r4/Mult  precision=Full  arith_type="Signed  (2's comp)"  n_bits=8  bin_pt=2  quantization=Truncate  overflow=Wrap  en=off  latency=latency  dbl_ovrd=off  use_behavioral_HDL=off  use_embedded=on  opt=Speed  optimum_pipeline=off  pipeline=on  use_rpm=off  placement_style=Rectangular shape  block_type=mult
      settings: infoedit=Hardware notes: To use the internal pipeline stage of the dedicated multiplier you must select 'Pipeline for maximum performance'.  xl_area=[0, 0, 0, 0, 0, 0, 0]  block_version=9.1.01
  Mult1 : xbsIndex_r4/Mult  precision=Full  arith_type="Signed  (2's comp)"  n_bits=8  bin_pt=2  quantization=Truncate  overflow=Wrap  en=off  latency=latency  dbl_ovrd=off  use_behavioral_HDL=off  use_embedded=on  opt=Speed  optimum_pipeline=off  pipeline=on  use_rpm=off  placement_style=Rectangular shape  block_type=mult
      settings: infoedit=Hardware notes: To use the internal pipeline stage of the dedicated multiplier you must select 'Pipeline for maximum performance'.  xl_area=[0, 0, 0, 0, 0, 0, 0]  block_version=9.1.01
  real : Outport
  imag : Outport  Port=2
  wires:
  cos/1 -> Mult/2
  sin/1 -> Mult1/2
  d/1 -> Mult/1, Mult1/1
  Mult/1 -> real/1
  Mult1/1 -> imag/1

== system casper_library/FFTs/Twiddle/coeff_gen ==
  br_coeff_gen : Subsystem  mask(br_coeff_gen){Coeffs=[0 1 2 3], StepPeriod=0, BitWidth=18, bram_latency=4}
      mask prompts: Coeffs "Coefficients: (0 to 2^(FFTSize-1)-1)"; StepPeriod "Step Period: (2^?)"; BitWidth "Bit Width:"; bram_latency "Latency:"
      mask init:
      | vlen = length(Coeffs);
  coeff_gen : Subsystem  BlockChoice=br_coeff_gen
      settings: TemplateBlock=self  MemberBlocks=br_coeff_gen,static_coeff_gen
  static_coeff_gen : Subsystem  mask(static_coeff_gen){Coeffs=0, BitWidth=18, bram_latency=4}
      mask prompts: Coeffs "Coefficients: (0 to 2^(FFTSize-1)-1)"; BitWidth "Bit Width:"; bram_latency "Latency:"

== system casper_library/FFTs/Twiddle/twiddle ==
  a : Inport
  b : Inport  Port=2
  sync : Inport  Port=3
  twiddle_coeff_0 : casper_library/FFTs/Twiddle/twiddle_coeff_0  SystemSampleTime=-1  BitWidth=18  add_latency=3  mult_latency=4  bram_latency=4
  a_re : Outport
  a_im : Outport  Port=2
  bw_re : Outport  Port=3
  bw_im : Outport  Port=4
  sync_out : Outport  Port=5
  wires:
  a/1 -> twiddle_coeff_0/1
  b/1 -> twiddle_coeff_0/2
  sync/1 -> twiddle_coeff_0/3
  twiddle_coeff_0/1 -> a_re/1
  twiddle_coeff_0/2 -> a_im/1
  twiddle_coeff_0/3 -> bw_re/1
  twiddle_coeff_0/4 -> bw_im/1
  twiddle_coeff_0/5 -> sync_out/1

== system casper_library/FFTs/Twiddle/twiddle_coeff_0 ==
  a : Inport
  b : Inport  Port=2
  sync : Inport  Port=3
  Delay : xbsIndex_r3/Delay  latency=mult_latency + add_latency + bram_latency  reg_retiming=off  explicit_period=off  period=1  en=off  accept_only_valid=off  init_zero=on  dbl_ovrd=off  show_param=off
      settings: xl_area=[0, 0, 0, 0, 0, 0, 0]
  Delay2 : xbsIndex_r3/Delay  latency=mult_latency + add_latency + bram_latency  reg_retiming=off  explicit_period=off  period=1  en=off  accept_only_valid=off  init_zero=on  dbl_ovrd=off  show_param=off
      settings: xl_area=[0, 0, 0, 0, 0, 0, 0]
  Delay3 : xbsIndex_r3/Delay  latency=mult_latency + add_latency + bram_latency  reg_retiming=off  explicit_period=off  period=1  en=off  accept_only_valid=off  init_zero=on  dbl_ovrd=off  show_param=off
      settings: xl_area=[0, 0, 0, 0, 0, 0, 0]
  c_to_ri : casper_library/Misc/c_to_ri  n_bits=BitWidth  bin_pt=BitWidth-1
      settings: AttributesFormatString=18_17 r/i
  c_to_ri1 : casper_library/Misc/c_to_ri  n_bits=BitWidth  bin_pt=BitWidth-1
      settings: AttributesFormatString=18_17 r/i
  a_re : Outport
  a_im : Outport  Port=2
  bw_re : Outport  Port=3
  bw_im : Outport  Port=4
  sync_out : Outport  Port=5
  wires:
  a/1 -> Delay/1
  sync/1 -> Delay2/1
  Delay2/1 -> sync_out/1
  b/1 -> Delay3/1
  Delay/1 -> c_to_ri/1
  c_to_ri/1 -> a_re/1
  c_to_ri/2 -> a_im/1
  c_to_ri1/1 -> bw_re/1
  c_to_ri1/2 -> bw_im/1
  Delay3/1 -> c_to_ri1/1

== system casper_library/FFTs/Twiddle/twiddle_coeff_1 ==
  a : Inport
  b : Inport  Port=2
  sync : Inport  Port=3
  Delay : xbsIndex_r3/Delay  latency=mult_latency + add_latency + bram_latency  reg_retiming=off  explicit_period=off  period=1  en=off  accept_only_valid=off  init_zero=on  dbl_ovrd=off  show_param=off
      settings: xl_area=[0, 0, 0, 0, 0, 0, 0]
  Delay2 : xbsIndex_r3/Delay  latency=mult_latency + add_latency + bram_latency  reg_retiming=off  explicit_period=off  period=1  en=off  accept_only_valid=off  init_zero=on  dbl_ovrd=off  show_param=off
      settings: xl_area=[0, 0, 0, 0, 0, 0, 0]
  Delay3 : xbsIndex_r3/Delay  latency=mult_latency + add_latency + bram_latency  reg_retiming=off  explicit_period=off  period=1  en=off  accept_only_valid=off  init_zero=on  dbl_ovrd=off  show_param=off
      settings: xl_area=[0, 0, 0, 0, 0, 0, 0]
  Negate : xbsIndex_r3/Negate  precision=User Defined  arith_type="Signed  (2's comp)"  n_bits=BitWidth  bin_pt=BitWidth-1  quantization=Truncate  overflow=Wrap  latency=mult_latency + add_latency + bram_latency  explicit_period=off  period=1  en=off  dbl_ovrd=off  use_core=on  show_param=off  use_rpm=on  gen_core=off
      settings: xl_area=[0, 0, 0, 0, 0, 0, 0]
  c_to_ri : casper_library/Misc/c_to_ri  n_bits=BitWidth  bin_pt=BitWidth-1
      settings: AttributesFormatString=18_17 r/i
  c_to_ri1 : casper_library/Misc/c_to_ri  n_bits=BitWidth  bin_pt=BitWidth-1
      settings: AttributesFormatString=18_17 r/i
  a_re : Outport
  a_im : Outport  Port=2
  bw_re : Outport  Port=3
  bw_im : Outport  Port=4
  sync_out : Outport  Port=5
  wires:
  c_to_ri/2 -> a_im/1
  c_to_ri/1 -> a_re/1
  Delay/1 -> c_to_ri/1
  b/1 -> c_to_ri1/1
  Delay2/1 -> sync_out/1
  sync/1 -> Delay2/1
  a/1 -> Delay/1
  c_to_ri1/1 -> Delay3/1
  Negate/1 -> bw_re/1
  c_to_ri1/2 -> Negate/1
  Delay3/1 -> bw_im/1

== system casper_library/FFTs/Twiddle/twiddle_general_3mult ==
  a : Inport
  b : Inport  Port=2
  sync : Inport  Port=3
  AddSub : xbsIndex_r3/AddSub  mode=Subtraction  precision=Full  arith_type="Signed  (2's comp)"  n_bits=BitWidth  bin_pt=BitWidth - 1  quantization="Round  (unbiased: +/- Inf)"  overflow=Wrap  latency=add_latency  explicit_period=off  period=1  use_carryin=off  use_carryout=off  en=off  dbl_ovrd=off  show_param=on  use_core=on  pipeline=on  use_rpm=on  gen_core=on
      settings: xl_area=[0, 0, 0, 0, 0, 0, 0]
  AddSub1 : xbsIndex_r3/AddSub  mode=Addition  precision=Full  arith_type="Signed  (2's comp)"  n_bits=BitWidth  bin_pt=BitWidth - 1  quantization="Round  (unbiased: +/- Inf)"  overflow=Wrap  latency=add_latency  explicit_period=off  period=1  use_carryin=off  use_carryout=off  en=off  dbl_ovrd=off  show_param=on  use_core=on  pipeline=on  use_rpm=on  gen_core=on
      settings: xl_area=[0, 0, 0, 0, 0, 0, 0]
  AddSub2 : xbsIndex_r3/AddSub  mode=Addition  precision=Full  arith_type="Signed  (2's comp)"  n_bits=BitWidth  bin_pt=BitWidth - 1  quantization="Round  (unbiased: +/- Inf)"  overflow=Wrap  latency=add_latency  explicit_period=off  period=1  use_carryin=off  use_carryout=off  en=off  dbl_ovrd=off  show_param=on  use_core=on  pipeline=on  use_rpm=on  gen_core=on
      settings: xl_area=[0, 0, 0, 0, 0, 0, 0]
  AddSub3 : xbsIndex_r3/AddSub  mode=Subtraction  precision=Full  arith_type="Signed  (2's comp)"  n_bits=BitWidth  bin_pt=BitWidth - 1  quantization="Round  (unbiased: +/- Inf)"  overflow=Wrap  latency=add_latency  explicit_period=off  period=1  use_carryin=off  use_carryout=off  en=off  dbl_ovrd=off  show_param=on  use_core=on  pipeline=on  use_rpm=on  gen_core=on
      settings: xl_area=[0, 0, 0, 0, 0, 0, 0]
  AddSub4 : xbsIndex_r3/AddSub  mode=Addition  precision=Full  arith_type="Signed  (2's comp)"  n_bits=BitWidth  bin_pt=BitWidth - 1  quantization="Round  (unbiased: +/- Inf)"  overflow=Wrap  latency=add_latency  explicit_period=off  period=1  use_carryin=off  use_carryout=off  en=off  dbl_ovrd=off  show_param=on  use_core=on  pipeline=on  use_rpm=on  gen_core=on
      settings: xl_area=[0, 0, 0, 0, 0, 0, 0]
  Convert : xbsIndex_r3/Convert  arith_type="Signed  (2's comp)"  n_bits=BitWidth  bin_pt=BitWidth-2  quantization=Truncate  overflow=Wrap  latency=0  explicit_period=off  period=1  dbl_ovrd=off  show_param=off  inserted_by_tool=off  pipeline=off
      settings: xl_area=[0, 0, 0, 0, 0, 0, 0]
  Convert1 : xbsIndex_r3/Convert  arith_type="Signed  (2's comp)"  n_bits=BitWidth  bin_pt=BitWidth-2  quantization=Truncate  overflow=Wrap  latency=0  explicit_period=off  period=1  dbl_ovrd=off  show_param=off  inserted_by_tool=off  pipeline=off
      settings: xl_area=[0, 0, 0, 0, 0, 0, 0]
  Convert2 : xbsIndex_r3/Convert  arith_type="Signed  (2's comp)"  n_bits=BitWidth  bin_pt=BitWidth-2  quantization=Truncate  overflow=Wrap  latency=0  explicit_period=off  period=1  dbl_ovrd=off  show_param=off  inserted_by_tool=off  pipeline=off
      settings: xl_area=[0, 0, 0, 0, 0, 0, 0]
  Convert3 : xbsIndex_r3/Convert  arith_type="Signed  (2's comp)"  n_bits=BitWidth + 3  bin_pt=BitWidth  quantization=Truncate  overflow=Wrap  latency=0  explicit_period=off  period=1  dbl_ovrd=off  show_param=off  inserted_by_tool=off  pipeline=off
      settings: xl_area=[0, 0, 0, 0, 0, 0, 0]
  Convert4 : xbsIndex_r3/Convert  arith_type="Signed  (2's comp)"  n_bits=BitWidth + 3  bin_pt=BitWidth  quantization=Truncate  overflow=Wrap  latency=0  explicit_period=off  period=1  dbl_ovrd=off  show_param=off  inserted_by_tool=off  pipeline=off
      settings: xl_area=[0, 0, 0, 0, 0, 0, 0]
  Convert5 : xbsIndex_r3/Convert  arith_type="Signed  (2's comp)"  n_bits=BitWidth + 3  bin_pt=BitWidth  quantization=Truncate  overflow=Wrap  latency=0  explicit_period=off  period=1  dbl_ovrd=off  show_param=off  inserted_by_tool=off  pipeline=off
      settings: xl_area=[0, 0, 0, 0, 0, 0, 0]
  Delay : xbsIndex_r3/Delay  latency=mult_latency + 2*add_latency + bram_latency  reg_retiming=off  explicit_period=off  period=1  en=off  accept_only_valid=off  init_zero=on  dbl_ovrd=off  show_param=off
      settings: xl_area=[0, 0, 0, 0, 0, 0, 0]
  Delay1 : xbsIndex_r3/Delay  latency=bram_latency  reg_retiming=off  explicit_period=off  period=1  en=off  accept_only_valid=off  init_zero=on  dbl_ovrd=off  show_param=off
      settings: xl_area=[0, 0, 0, 0, 0, 0, 0]
  Delay2 : xbsIndex_r3/Delay  latency=mult_latency + 2*add_latency + bram_latency  reg_retiming=off  explicit_period=off  period=1  en=off  accept_only_valid=off  init_zero=on  dbl_ovrd=off  show_param=off
      settings: xl_area=[0, 0, 0, 0, 0, 0, 0]
  Delay3 : xbsIndex_r3/Delay  latency=add_latency  reg_retiming=off  explicit_period=off  period=1  en=off  accept_only_valid=off  init_zero=on  dbl_ovrd=off  show_param=off
      settings: xl_area=[0, 0, 0, 0, 0, 0, 0]
  Delay4 : xbsIndex_r3/Delay  latency=add_latency  reg_retiming=off  explicit_period=off  period=1  en=off  accept_only_valid=off  init_zero=on  dbl_ovrd=off  show_param=off
      settings: xl_area=[0, 0, 0, 0, 0, 0, 0]
  Delay5 : xbsIndex_r3/Delay  latency=add_latency  reg_retiming=off  explicit_period=off  period=1  en=off  accept_only_valid=off  init_zero=on  dbl_ovrd=off  show_param=off
      settings: xl_area=[0, 0, 0, 0, 0, 0, 0]
  Mult : xbsIndex_r3/Mult  precision=Full  arith_type="Signed  (2's comp)"  n_bits=BitWidth  bin_pt=BitWidth-1  quantization="Round  (unbiased: +/- Inf)"  overflow=Wrap  latency=mult_latency  explicit_period=off  period=1  en=off  dbl_ovrd=off  show_param=on  mult_type=Parallel  oversample=2  use_embedded=on  pipeline=on  use_rpm=on  placement_style=Rectangular Shape  gen_core=on
      settings: xl_area=[0, 0, 0, 0, 0, 0, 0]
  Mult1 : xbsIndex_r3/Mult  precision=Full  arith_type="Signed  (2's comp)"  n_bits=BitWidth  bin_pt=BitWidth-1  quantization="Round  (unbiased: +/- Inf)"  overflow=Wrap  latency=mult_latency  explicit_period=off  period=1  en=off  dbl_ovrd=off  show_param=on  mult_type=Parallel  oversample=2  use_embedded=on  pipeline=on  use_rpm=on  placement_style=Rectangular Shape  gen_core=on
      settings: xl_area=[0, 0, 0, 0, 0, 0, 0]
  Mult2 : xbsIndex_r3/Mult  precision=Full  arith_type="Signed  (2's comp)"  n_bits=BitWidth  bin_pt=BitWidth-1  quantization="Round  (unbiased: +/- Inf)"  overflow=Wrap  latency=mult_latency  explicit_period=off  period=1  en=off  dbl_ovrd=off  show_param=on  mult_type=Parallel  oversample=2  use_embedded=on  pipeline=on  use_rpm=on  placement_style=Rectangular Shape  gen_core=on
      settings: xl_area=[0, 0, 0, 0, 0, 0, 0]
  c_to_ri1 : casper_library/Misc/c_to_ri  n_bits=BitWidth  bin_pt=BitWidth-1
      settings: AttributesFormatString=18_17 r/i
  c_to_ri2 : casper_library/Misc/c_to_ri  n_bits=BitWidth  bin_pt=BitWidth-1
      settings: AttributesFormatString=18_17 r/i
  c_to_ri3 : casper_library/Misc/c_to_ri  n_bits=BitWidth  bin_pt=BitWidth-1
      settings: AttributesFormatString=18_17 r/i
  coeff_gen : Subsystem  BlockChoice=static_coeff_gen
      link override br_coeff_gen: Coeffs=Coeffs  StepPeriod=StepPeriod  BitWidth=BitWidth  bram_latency=bram_latency
      link override static_coeff_gen: Coeffs=Coeffs  n_bits=BitWidth  latency=bram_latency  BitWidth=BitWidth  bram_latency=bram_latency
      link override static_coeff_gen/Constant: equ=P=C
      link override static_coeff_gen/Constant1: equ=P=C
      settings: AttributesFormatString=%<BlockChoice>  TemplateBlock=casper_library/FFTs/Twiddle/coeff_gen/coeff_gen  MemberBlocks=br_coeff_gen,static_coeff_gen
  a_re : Outport
  a_im : Outport  Port=2
  bw_re : Outport  Port=3
  bw_im : Outport  Port=4
  sync_out : Outport  Port=5
  wires:
  Convert5/1 -> AddSub4/2
  Convert4/1 -> AddSub/2
  Convert3/1 -> AddSub4/1, AddSub/1
  AddSub4/1 -> bw_im/1
  AddSub/1 -> bw_re/1
  Mult2/1 -> Convert5/1
  Mult1/1 -> Convert4/1
  Mult/1 -> Convert3/1
  Delay3/1 -> Mult2/1
  Delay5/1 -> Mult/2
  Delay4/1 -> Mult1/1
  Convert2/1 -> Mult2/2
  Convert1/1 -> Mult1/2
  Convert/1 -> Mult/1
  AddSub1/1 -> Convert/1
  AddSub2/1 -> Convert1/1
  AddSub3/1 -> Convert2/1
  c_to_ri2/2 -> AddSub3/1, AddSub2/2
  c_to_ri2/1 -> Delay5/1, AddSub3/2, AddSub2/1
  c_to_ri3/2 -> Delay4/1, AddSub1/2
  c_to_ri3/1 -> Delay3/1, AddSub1/1
  coeff_gen/1(w) -> c_to_ri2/1
  Delay1/1 -> c_to_ri3/1
  b/1 -> Delay1/1
  c_to_ri1/2 -> a_im/1
  c_to_ri1/1 -> a_re/1
  Delay/1 -> c_to_ri1/1
  a/1 -> Delay/1
  sync/1 -> Delay2/1, coeff_gen/1(rst)
  Delay2/1 -> sync_out/1
